simulink model "torqueWalking"  (Simulink 8.9)
settings: Solver=FixedStepDiscrete  StartTime=0.0  StopTime=Config.t_end  FixedStep=Config.t_step  RelTol=1e-3  EnableMultiTasking=on
InitFcn:
  | cd(fileparts(which(bdroot)));
  | initTorqueWalking;
StopFcn:
  | cd(fileparts(which(bdroot)));
  | outputTorqueWalking
values from neighbouring files (symbols this model uses):
  weights = [1 1 1 1 0.001 0.0001]    [inputWeights.mat]
undefined symbols (not defined in the file or in its folder): biasVectorConstraint_feet, Config, ConstraintMatrix_feet, DiscIntNeverNeededParam, Gains, ROBOT_DOF, Sat
libraries: WBToolboxLibrary x114
(part 3 of 4)

== system torqueWalking/Robot State and References/Smooth References /Smooth Reference Positions ==
  pos_CoM_des : Inport
  pos_LFoot_des : Inport  Port=2
  pos_RFoot_des : Inport  Port=3
  s_des : Inport  Port=4
  pos_LHand_des : Inport  Port=5
  pos_RHand_des : Inport  Port=6
  state : Inport  Port=7
  Configure Settling Times : MATLAB Function  TreatAsAtomicUnit=on
  Matrix Concatenate1 : Concatenate  NumInputs=3  Mode=Multidimensional array  ConcatenateDimension=2
  Matrix Concatenate{2..3,5..6} (4 alike) : Concatenate  NumInputs=4  Mode=Multidimensional array  ConcatenateDimension=2
  Matrix Concatenate4 : Concatenate  NumInputs=3  Mode=Multidimensional array  ConcatenateDimension=2
  Minimum Jerk Trajectory Generator{,1..3,5..6} (6 alike) : WBToolboxLibrary/Utilities/Minimum Jerk Trajectory Generator  externalSettlingTime=on  settlingTime=3  sampleTime=Config.t_step  resetOnSettlingTime=off  firstDerivatives=on  secondDerivatives=on  explicitInitialValue=off
  Settling time1 : Constant  Value=zeros(3,2)
  smooth_references_CoM : Outport
  smooth_pos_vel_acc_LFoot : Outport  Port=2
  smooth_pos_vel_acc_RFoot : Outport  Port=3
  smooth_pos_vel_acc_LHand : Outport  Port=4
  smooth_pos_vel_acc_RHand : Outport  Port=5
  smooth_references_s : Outport  Port=6
  wires:
  Minimum Jerk Trajectory Generator2/2 -> Matrix Concatenate3/2
  pos_RFoot_des/1 -> Minimum Jerk Trajectory Generator3/1
  s_des/1 -> Minimum Jerk Trajectory Generator1/1
  Minimum Jerk Trajectory Generator2/3 -> Matrix Concatenate3/3
  Minimum Jerk Trajectory Generator2/1 -> Matrix Concatenate3/1
  Matrix Concatenate4/1 -> smooth_references_CoM/1
  pos_CoM_des/1 -> Minimum Jerk Trajectory Generator/1
  Minimum Jerk Trajectory Generator/3 -> Matrix Concatenate4/3
  Minimum Jerk Trajectory Generator/2 -> Matrix Concatenate4/2
  Minimum Jerk Trajectory Generator3/3 -> Matrix Concatenate2/3
  Matrix Concatenate3/1 -> smooth_pos_vel_acc_LFoot/1
  Matrix Concatenate2/1 -> smooth_pos_vel_acc_RFoot/1
  Minimum Jerk Trajectory Generator/1 -> Matrix Concatenate4/1
  Minimum Jerk Trajectory Generator3/2 -> Matrix Concatenate2/2
  pos_LFoot_des/1 -> Minimum Jerk Trajectory Generator2/1
  Minimum Jerk Trajectory Generator3/1 -> Matrix Concatenate2/1
  state/1 -> Configure Settling Times/1(state)
  Configure Settling Times/1(smoothingTime_CoM) -> Minimum Jerk Trajectory Generator/2
  Configure Settling Times/2(smoothingTime_LFoot) -> Minimum Jerk Trajectory Generator2/2
  Configure Settling Times/3(smoothingTime_RFoot) -> Minimum Jerk Trajectory Generator3/2
  Configure Settling Times/4(smoothingTime_joints) -> Minimum Jerk Trajectory Generator1/2
  Configure Settling Times/6(smoothingTime_RHand) -> Minimum Jerk Trajectory Generator6/2
  Configure Settling Times/5(smoothingTime_LHand) -> Minimum Jerk Trajectory Generator5/2
  Minimum Jerk Trajectory Generator6/1 -> Matrix Concatenate5/1
  Settling time1/1 -> Matrix Concatenate3/4, Matrix Concatenate2/4, Matrix Concatenate6/4, Matrix Concatenate5/4
  Minimum Jerk Trajectory Generator6/2 -> Matrix Concatenate5/2
  Matrix Concatenate5/1 -> smooth_pos_vel_acc_RHand/1
  Matrix Concatenate6/1 -> smooth_pos_vel_acc_LHand/1
  Minimum Jerk Trajectory Generator6/3 -> Matrix Concatenate5/3
  Minimum Jerk Trajectory Generator5/1 -> Matrix Concatenate6/1
  Minimum Jerk Trajectory Generator5/3 -> Matrix Concatenate6/3
  pos_RHand_des/1 -> Minimum Jerk Trajectory Generator6/1
  pos_LHand_des/1 -> Minimum Jerk Trajectory Generator5/1
  Minimum Jerk Trajectory Generator5/2 -> Matrix Concatenate6/2
  Matrix Concatenate1/1 -> smooth_references_s/1
  Minimum Jerk Trajectory Generator1/3 -> Matrix Concatenate1/3
  Minimum Jerk Trajectory Generator1/2 -> Matrix Concatenate1/2
  Minimum Jerk Trajectory Generator1/1 -> Matrix Concatenate1/1

== system torqueWalking/Robot State and References/State Machines/Compute Feet to Base Link Transforms ==
  s : Inport
  w_H_base_fixed : Inport  Port=2
  IMU port : Inport  Port=3
  Constant : Constant  Value=Config.LFoot_in_contact_at0
  "LFoot to base link transform " : Subsystem
  LFoot to world transform (fixed base) : WBToolboxLibrary/wholeBodyModel/Kinematics/Forward Kinematics  frameName=Frames.LEFT_FOOT  robotName=WBT_robotName  localName=WBT_modelName  wbiFile=WBT_wbiFilename  wbiList=WBT_wbiList
  RFoot to base link transform : Subsystem
  RFoot to world transform (fixed base) : WBToolboxLibrary/wholeBodyModel/Kinematics/Forward Kinematics  frameName=Frames.RIGHT_FOOT  robotName=WBT_robotName  localName=WBT_modelName  wbiFile=WBT_wbiFilename  wbiList=WBT_wbiList
  Switch6 : Switch  Criteria=u2 > Threshold
  fixed_link_H_b : Outport
  LFoot_H_b : Outport  Port=2
  RFoot_H_b : Outport  Port=3
  wires:
  RFoot to world transform (fixed base)/1 -> RFoot to base link transform/3(w_H_link)
  s/1 -> RFoot to base link transform/1(s), "LFoot to base link transform "/1(s), RFoot to world transform (fixed base)/2, LFoot to world transform (fixed base)/2
  LFoot to world transform (fixed base)/1 -> "LFoot to base link transform "/3(w_H_link)
  w_H_base_fixed/1 -> RFoot to base link transform/4(w_H_base_fixed), RFoot to world transform (fixed base)/1, "LFoot to base link transform "/4(w_H_base_fixed), LFoot to world transform (fixed base)/1
  IMU port/1 -> RFoot to base link transform/2(inertial), "LFoot to base link transform "/2(inertial)
  RFoot to base link transform/1(link_H_b) -> Switch6/3, RFoot_H_b/1
  Constant/1 -> Switch6/2
  "LFoot to base link transform "/1(link_H_b) -> LFoot_H_b/1, Switch6/1
  Switch6/1 -> fixed_link_H_b/1

== system torqueWalking/Robot State and References/State Machines/Compute State Velocity ==
  s : Inport
  w_H_b : Inport  Port=2
  "feetInContact " : Inport  Port=3
  Compute Base Velocity : MATLAB Function  TreatAsAtomicUnit=on
  Feet Jacobians : Subsystem
  Get Estimate : WBToolboxLibrary/wholeBodyStates/Get Estimate  estimateType=Joints Velocity  robotName=WBT_robotName  localName=WBT_modelName  wbiFile=WBT_wbiFilename  wbiList=WBT_wbiList
  Mux : Mux  Inputs=2
  nu : Outport
  wires:
  Get Estimate/1 -> Mux/2, Compute Base Velocity/4(sDot)
  Mux/1 -> nu/1
  "feetInContact "/1 -> Compute Base Velocity/3(feetInContact)
  Compute Base Velocity/1(nu_b) -> Mux/1
  s/1 -> Feet Jacobians/1(s)
  w_H_b/1 -> Feet Jacobians/2(w_H_b)
  Feet Jacobians/1(J_LFoot) -> Compute Base Velocity/1(J_LeftFoot)
  Feet Jacobians/2(J_RFoot) -> Compute Base Velocity/2(J_RightFoot)

== system torqueWalking/Robot State and References/State Machines/Select the Current State and References ==
  s : Inport
  fixed_link_H_b : Inport  Port=2
  LFoot_H_b : Inport  Port=3
  RFoot_H_b : Inport  Port=4
  Clock : Clock
  STATE MACHINES : MATLAB Function  TreatAsAtomicUnit=on
  holder {1..7} (7 alike) : WBToolboxLibrary/Utilities/holder 
  left_foot_wrench : WBToolboxLibrary/Utilities/Yarp Read  portName=Ports.LEFT_FOOT_EXT_WRENCH  signalSize=6  blocking=off  timestamp=off  autoconnect=on  errorOnConnection=on
  right_foot_wrench : WBToolboxLibrary/Utilities/Yarp Read  portName=Ports.RIGHT_FOOT_EXT_WRENCH  signalSize=6  blocking=off  timestamp=off  autoconnect=on  errorOnConnection=on
  task position and orientation : Subsystem
  w_H_b : Outport
  feetInContact : Outport  Port=2
  state : Outport  Port=3
  references_CoM : Outport  Port=4
  references_LFoot : Outport  Port=5
  references_RFoot : Outport  Port=6
  references_rot_task : Outport  Port=7
  references_LHand : Outport  Port=8
  references_RHand : Outport  Port=9
  references_s : Outport  Port=10
  wires:
  STATE MACHINES/3(references_LFoot) -> references_LFoot/1
  task position and orientation/2(w_H_l_sole) -> holder 2/1
  holder 3/1 -> STATE MACHINES/4(w_H_RFoot_0)
  STATE MACHINES/5(references_rot_task) -> references_rot_task/1
  STATE MACHINES/4(references_RFoot) -> references_RFoot/1
  s/1 -> holder 5/1, task position and orientation/1(s)
  holder 4/1 -> STATE MACHINES/5(w_H_rot_task_0)
  task position and orientation/1(w_H_CoM) -> holder 1/1
  holder 2/1 -> STATE MACHINES/3(w_H_LFoot_0)
  task position and orientation/4(w_H_rot_task) -> holder 4/1
  STATE MACHINES/1(state) -> state/1
  STATE MACHINES/8(feetInContact) -> feetInContact/1
  task position and orientation/3(w_H_r_sole) -> holder 3/1
  Clock/1 -> STATE MACHINES/10(t)
  STATE MACHINES/9(references_s) -> references_s/1
  STATE MACHINES/2(references_CoM) -> references_CoM/1
  holder 1/1 -> STATE MACHINES/2(w_H_CoM_0)
  holder 5/1 -> STATE MACHINES/1(s_0)
  STATE MACHINES/10(w_H_b) -> w_H_b/1
  fixed_link_H_b/1 -> task position and orientation/2(w_H_b)
  LFoot_H_b/1 -> STATE MACHINES/8(LFoot_H_b)
  RFoot_H_b/1 -> STATE MACHINES/9(RFoot_H_b)
  left_foot_wrench/1 -> STATE MACHINES/11(LFoot_wrench)
  right_foot_wrench/1 -> STATE MACHINES/12(RFoot_wrench)
  holder 6/1 -> STATE MACHINES/6(w_H_LHand_0)
  task position and orientation/5(w_H_l_hand) -> holder 6/1
  task position and orientation/6(w_H_r_hand) -> holder 7/1
  holder 7/1 -> STATE MACHINES/7(w_H_RHand_0)
  STATE MACHINES/6(references_LHand) -> references_LHand/1
  STATE MACHINES/7(references_RHand) -> references_RHand/1

== system torqueWalking/Visualization/Cartesian Tasks/Rotation Error Left Foot ==
  w_R_RFoot : Inport
  w_R_RFoot_des : Inport  Port=2
  Constant : Constant  Value=eye(3)
  Demux : Demux  Outputs=3
  Permute Dimensions1 : PermuteDimensions
  Permute Dimensions2 : PermuteDimensions
  Product : Product  Multiplication=Matrix(*)
  Product2 : Product  Multiplication=Matrix(*)
  Reshape2 : Reshape
  Selector : Selector  InputPortWidth=9  IndexOptions=Index vector (dialog)  Indices=[1 5 9]  OutputSizes=1
  Sum : Sum  Inputs=|-+
  Sum of Elements : Sum  Inputs=+++
  |1-R^T*RDes|^2 : Outport
  wires:
  w_R_RFoot_des/1 -> Product2/2
  Product2/1 -> Sum/1
  w_R_RFoot/1 -> Permute Dimensions2/1
  Sum/1 -> Product/2, Permute Dimensions1/1
  Permute Dimensions2/1 -> Product2/1
  Constant/1 -> Sum/2
  Permute Dimensions1/1 -> Product/1
  Product/1 -> Reshape2/1
  Reshape2/1 -> Selector/1
  Selector/1 -> Demux/1
  Demux/1 -> Sum of Elements/1
  Demux/2 -> Sum of Elements/2
  Demux/3 -> Sum of Elements/3
  Sum of Elements/1 -> |1-R^T*RDes|^2/1

== system torqueWalking/Visualization/Cartesian Tasks/Rotation Error Right Foot ==
  w_R_LFoot : Inport
  w_R_LFoot_des : Inport  Port=2
  Constant : Constant  Value=eye(3)
  Demux : Demux  Outputs=3
  Permute Dimensions1 : PermuteDimensions
  Permute Dimensions2 : PermuteDimensions
  Product : Product  Multiplication=Matrix(*)
  Product2 : Product  Multiplication=Matrix(*)
  Reshape2 : Reshape
  Selector : Selector  InputPortWidth=9  IndexOptions=Index vector (dialog)  Indices=[1 5 9]  OutputSizes=1
  Sum : Sum  Inputs=|-+
  Sum of Elements : Sum  Inputs=+++
  |1-R^T*RDes|^2 : Outport
  wires:
  w_R_LFoot_des/1 -> Product2/2
  Product2/1 -> Sum/1
  w_R_LFoot/1 -> Permute Dimensions2/1
  Sum/1 -> Product/2, Permute Dimensions1/1
  Permute Dimensions2/1 -> Product2/1
  Constant/1 -> Sum/2
  Permute Dimensions1/1 -> Product/1
  Product/1 -> Reshape2/1
  Reshape2/1 -> Selector/1
  Selector/1 -> Demux/1
  Demux/1 -> Sum of Elements/1
  Demux/2 -> Sum of Elements/2
  Demux/3 -> Sum of Elements/3
  Sum of Elements/1 -> |1-R^T*RDes|^2/1

== system torqueWalking/Visualization/Cartesian Tasks/Rotation Error Rotational Task ==
  w_R_rot_task : Inport
  w_R_rot_task_des : Inport  Port=2
  Constant : Constant  Value=eye(3)
  Demux : Demux  Outputs=3
  Permute Dimensions1 : PermuteDimensions
  Permute Dimensions2 : PermuteDimensions
  Product : Product  Multiplication=Matrix(*)
  Product2 : Product  Multiplication=Matrix(*)
  Reshape2 : Reshape
  Selector : Selector  InputPortWidth=9  IndexOptions=Index vector (dialog)  Indices=[1 5 9]  OutputSizes=1
  Sum : Sum  Inputs=|-+
  Sum of Elements : Sum  Inputs=+++
  |1-R^T*RDes|^2 : Outport
  wires:
  w_R_rot_task_des/1 -> Product2/2
  Product2/1 -> Sum/1
  w_R_rot_task/1 -> Permute Dimensions2/1
  Sum/1 -> Product/2, Permute Dimensions1/1
  Permute Dimensions2/1 -> Product2/1
  Constant/1 -> Sum/2
  Permute Dimensions1/1 -> Product/1
  Product/1 -> Reshape2/1
  Reshape2/1 -> Selector/1
  Selector/1 -> Demux/1
  Demux/1 -> Sum of Elements/1
  Demux/2 -> Sum of Elements/2
  Demux/3 -> Sum of Elements/3
  Sum of Elements/1 -> |1-R^T*RDes|^2/1

== system torqueWalking/Visualization/Orientation Tasks References/Rotation Error Left Foot ==
  w_R_LFoot : Inport
  w_R_LFoot_des : Inport  Port=2
  Constant : Constant  Value=eye(3)
  Demux : Demux  Outputs=3
  Permute Dimensions1 : PermuteDimensions
  Permute Dimensions2 : PermuteDimensions
  Product : Product  Multiplication=Matrix(*)
  Product2 : Product  Multiplication=Matrix(*)
  Reshape2 : Reshape
  Selector : Selector  InputPortWidth=9  IndexOptions=Index vector (dialog)  Indices=[1 5 9]  OutputSizes=1
  Sum : Sum  Inputs=|-+
  Sum of Elements : Sum  Inputs=+++
  |1-R^T*RDes|^2 : Outport
  wires:
  w_R_LFoot_des/1 -> Product2/2
  Product2/1 -> Sum/1
  w_R_LFoot/1 -> Permute Dimensions2/1
  Sum/1 -> Product/2, Permute Dimensions1/1
  Permute Dimensions2/1 -> Product2/1
  Constant/1 -> Sum/2
  Permute Dimensions1/1 -> Product/1
  Product/1 -> Reshape2/1
  Reshape2/1 -> Selector/1
  Selector/1 -> Demux/1
  Demux/1 -> Sum of Elements/1
  Demux/2 -> Sum of Elements/2
  Demux/3 -> Sum of Elements/3
  Sum of Elements/1 -> |1-R^T*RDes|^2/1

== system torqueWalking/Visualization/Orientation Tasks References/Rotation Error Right Foot ==
  w_R_RFoot : Inport
  w_R_RFoot_des : Inport  Port=2
  Constant : Constant  Value=eye(3)
  Demux : Demux  Outputs=3
  Permute Dimensions1 : PermuteDimensions
  Permute Dimensions2 : PermuteDimensions
  Product : Product  Multiplication=Matrix(*)
  Product2 : Product  Multiplication=Matrix(*)
  Reshape2 : Reshape
  Selector : Selector  InputPortWidth=9  IndexOptions=Index vector (dialog)  Indices=[1 5 9]  OutputSizes=1
  Sum : Sum  Inputs=|-+
  Sum of Elements : Sum  Inputs=+++
  |1-R^T*RDes|^2 : Outport
  wires:
  w_R_RFoot_des/1 -> Product2/2
  Product2/1 -> Sum/1
  w_R_RFoot/1 -> Permute Dimensions2/1
  Sum/1 -> Product/2, Permute Dimensions1/1
  Permute Dimensions2/1 -> Product2/1
  Constant/1 -> Sum/2
  Permute Dimensions1/1 -> Product/1
  Product/1 -> Reshape2/1
  Reshape2/1 -> Selector/1
  Selector/1 -> Demux/1
  Demux/1 -> Sum of Elements/1
  Demux/2 -> Sum of Elements/2
  Demux/3 -> Sum of Elements/3
  Sum of Elements/1 -> |1-R^T*RDes|^2/1

== system torqueWalking/Visualization/Orientation Tasks References/Rotation Error Rotational Task ==
  w_R_rot_task : Inport
  w_R_rot_task_des : Inport  Port=2
  Constant : Constant  Value=eye(3)
  Demux : Demux  Outputs=3
  Permute Dimensions1 : PermuteDimensions
  Permute Dimensions2 : PermuteDimensions
  Product : Product  Multiplication=Matrix(*)
  Product2 : Product  Multiplication=Matrix(*)
  Reshape2 : Reshape
  Selector : Selector  InputPortWidth=9  IndexOptions=Index vector (dialog)  Indices=[1 5 9]  OutputSizes=1
  Sum : Sum  Inputs=|-+
  Sum of Elements : Sum  Inputs=+++
  |1-R^T*RDes|^2 : Outport
  wires:
  w_R_rot_task_des/1 -> Product2/2
  Product2/1 -> Sum/1
  w_R_rot_task/1 -> Permute Dimensions2/1
  Sum/1 -> Product/2, Permute Dimensions1/1
  Permute Dimensions2/1 -> Product2/1
  Constant/1 -> Sum/2
  Permute Dimensions1/1 -> Product/1
  Product/1 -> Reshape2/1
  Reshape2/1 -> Selector/1
  Selector/1 -> Demux/1
  Demux/1 -> Sum of Elements/1
  Demux/2 -> Sum of Elements/2
  Demux/3 -> Sum of Elements/3
  Sum of Elements/1 -> |1-R^T*RDes|^2/1

== system torqueWalking/Dynamics and Kinematics/Compute Dynamic and Kinematic Quantities/Mass Matrix and Bias Forces/Add motors reflected inertias ==
  M : Inport
  Add motor reflected inertias : MATLAB Function  TreatAsAtomicUnit=on
  M_with_motor_inertia : Outport
  wires:
  M/1 -> Add motor reflected inertias/1(M)
  Add motor reflected inertias/1(M_with_inertia) -> M_with_motor_inertia/1

== system torqueWalking/Dynamics and Kinematics/Initial Conditions/compute state velocity/Feet Jacobians ==
  s : Inport
  w_H_b : Inport  Port=2
  Jacobian LFoot : WBToolboxLibrary/wholeBodyModel/Jacobians/Jacobian  frameName=Frames.LEFT_FOOT  robotName=WBT_robotName  localName=WBT_modelName  wbiFile=WBT_wbiFilename  wbiList=WBT_wbiList
  Jacobian RFoot : WBToolboxLibrary/wholeBodyModel/Jacobians/Jacobian  frameName=Frames.RIGHT_FOOT  robotName=WBT_robotName  localName=WBT_modelName  wbiFile=WBT_wbiFilename  wbiList=WBT_wbiList
  J_LFoot : Outport
  J_RFoot : Outport  Port=2
  wires:
  Jacobian LFoot/1 -> J_LFoot/1
  Jacobian RFoot/1 -> J_RFoot/1
  w_H_b/1 -> Jacobian RFoot/1, Jacobian LFoot/1
  s/1 -> Jacobian LFoot/2, Jacobian RFoot/2

== system torqueWalking/Dynamics and Kinematics/Inverse Kinematics/ComputeTasksPoseAndVelocity/Task position and orientation ==
  s : Inport
  w_H_b : Inport  Port=2
  CoM : WBToolboxLibrary/wholeBodyModel/Kinematics/Forward Kinematics  frameName=Frames.COM  robotName=WBT_robotName  localName=WBT_modelName  wbiFile=WBT_wbiFilename  wbiList=WBT_wbiList
  LFoot : WBToolboxLibrary/wholeBodyModel/Kinematics/Forward Kinematics  frameName=Frames.LEFT_FOOT  robotName=WBT_robotName  localName=WBT_modelName  wbiFile=WBT_wbiFilename  wbiList=WBT_wbiList
  LFoot1 : WBToolboxLibrary/wholeBodyModel/Kinematics/Forward Kinematics  frameName=Frames.LEFT_HAND  robotName=WBT_robotName  localName=WBT_modelName  wbiFile=WBT_wbiFilename  wbiList=WBT_wbiList
  RFoot : WBToolboxLibrary/wholeBodyModel/Kinematics/Forward Kinematics  frameName=Frames.RIGHT_FOOT  robotName=WBT_robotName  localName=WBT_modelName  wbiFile=WBT_wbiFilename  wbiList=WBT_wbiList
  RFoot1 : WBToolboxLibrary/wholeBodyModel/Kinematics/Forward Kinematics  frameName=Frames.RIGHT_HAND  robotName=WBT_robotName  localName=WBT_modelName  wbiFile=WBT_wbiFilename  wbiList=WBT_wbiList
  rotational task : WBToolboxLibrary/wholeBodyModel/Kinematics/Forward Kinematics  frameName=Frames.ROT_TASK_LINK  robotName=WBT_robotName  localName=WBT_modelName  wbiFile=WBT_wbiFilename  wbiList=WBT_wbiList
  w_H_CoM : Outport
  w_H_l_sole : Outport  Port=2
  w_H_r_sole : Outport  Port=3
  w_H_rot_task : Outport  Port=4
  w_H_l_hand : Outport  Port=5
  w_H_r_hand : Outport  Port=6
  wires:
  s/1 -> rotational task/2, RFoot1/2, LFoot1/2, RFoot/2, LFoot/2, CoM/2
  w_H_b/1 -> LFoot1/1, RFoot1/1, rotational task/1, CoM/1, LFoot/1, RFoot/1
  CoM/1 -> w_H_CoM/1
  LFoot/1 -> w_H_l_sole/1
  RFoot/1 -> w_H_r_sole/1
  rotational task/1 -> w_H_rot_task/1
  RFoot1/1 -> w_H_r_hand/1
  LFoot1/1 -> w_H_l_hand/1

== system torqueWalking/Dynamics and Kinematics/Inverse Kinematics/QP-Based Inverse Kinematics/QP Solver (inverse kinematics) ==
  Hessian : Inport
  gradient : Inport  Port=2
  ConstraintMatrix : Inport  Port=3
  biasVectorConstraint : Inport  Port=4
  QPSolver : M-S-Function  FunctionName=QPInverseKinematics  Parameters=ROBOT_DOF, Sat, Config
  nuDot : Outport
  ExitFlagQP : Outport  Port=2
  wires:
  QPSolver/1 -> nuDot/1
  QPSolver/2 -> ExitFlagQP/1
  Hessian/1 -> QPSolver/1
  gradient/1 -> QPSolver/2
  biasVectorConstraint/1 -> QPSolver/4
  ConstraintMatrix/1 -> QPSolver/3

== system torqueWalking/Dynamics and Kinematics/Inverse Kinematics/QP-Based Inverse Kinematics/inverse kinematics integration ==
  nuDot : Inport
  nu_0 : Inport  Port=2
  q_0 : Inport  Port=3
  Compute Base Pose Derivative : MATLAB Function  TreatAsAtomicUnit=on
  Demux : Demux  Outputs=[7;ROBOT_DOF]
  Demux1 : Demux  Outputs=[6; ROBOT_DOF]
  Demux2 : Demux  Outputs=[16; ROBOT_DOF]
  Integrate nu : DiscreteIntegrator  InitialConditionSource=external  SampleTime=Config.t_step  ICPrevOutput=DiscIntNeverNeededParam  ICPrevScaledInput=DiscIntNeverNeededParam
  Integrate nuDot : DiscreteIntegrator  InitialConditionSource=external  SampleTime=Config.t_step  ICPrevOutput=DiscIntNeverNeededParam  ICPrevScaledInput=DiscIntNeverNeededParam
  Matrix Concatenate : Concatenate  NumInputs=3  Mode=Multidimensional array  ConcatenateDimension=2
  Mux : Mux  Inputs=2
  Mux1 : Mux  Inputs=2
  Mux2 : Mux  Inputs=2
  Reshape : Reshape
  Reshape1 : Reshape  OutputDimensionality=Customize  OutputDimensions=[4;4]
  Rewrite Base Pose as pos+quat : MATLAB Function  TreatAsAtomicUnit=on
  Rewrite Base Pose as transformation matrix : MATLAB Function  TreatAsAtomicUnit=on
  Selector3 : Selector  InputPortWidth=ROBOT_DOF+6  IndexOptions=Index vector (dialog)  Indices=[7:ROBOT_DOF+6]  OutputSizes=1
  Selector4 : Selector  InputPortWidth=ROBOT_DOF+6  IndexOptions=Index vector (dialog)  Indices=[7:ROBOT_DOF+6]  OutputSizes=1
  nu : Outport
  q : Outport  Port=2
  s_sDot_sDDot_des : Outport  Port=3
  wires:
  nu_0/1 -> Integrate nuDot/2
  nuDot/1 -> Selector4/1, Integrate nuDot/1
  Demux/1 -> Rewrite Base Pose as transformation matrix/1(pose_b), Compute Base Pose Derivative/1(pose_b)
  Integrate nu/1 -> Demux/1
  Compute Base Pose Derivative/1(pose_bDot) -> Mux/1
  Demux1/2 -> Mux/2
  Matrix Concatenate/1 -> s_sDot_sDDot_des/1
  Selector3/1 -> Matrix Concatenate/2
  Selector4/1 -> Matrix Concatenate/3
  Demux/2 -> Matrix Concatenate/1, Mux1/2
  Mux/1 -> Integrate nu/1
  Integrate nuDot/1 -> Selector3/1, nu/1, Demux1/1
  Rewrite Base Pose as transformation matrix/1(w_H_b) -> Reshape/1
  Reshape/1 -> Mux1/1
  Mux1/1 -> q/1
  Demux1/1 -> Compute Base Pose Derivative/2(nu_b)
  q_0/1 -> Demux2/1
  Demux2/1 -> Reshape1/1
  Reshape1/1 -> Rewrite Base Pose as pos+quat/1(w_H_b_0)
  Rewrite Base Pose as pos+quat/1(pose_b_0) -> Mux2/1
  Demux2/2 -> Mux2/2
  Mux2/1 -> Integrate nu/2

== system torqueWalking/Dynamics and Kinematics/Task Accelerations/ComputeTasksPoseAndVelocity/Task position and orientation ==
  s : Inport
  w_H_b : Inport  Port=2
  CoM : WBToolboxLibrary/wholeBodyModel/Kinematics/Forward Kinematics  frameName=Frames.COM  robotName=WBT_robotName  localName=WBT_modelName  wbiFile=WBT_wbiFilename  wbiList=WBT_wbiList
  LFoot : WBToolboxLibrary/wholeBodyModel/Kinematics/Forward Kinematics  frameName=Frames.LEFT_FOOT  robotName=WBT_robotName  localName=WBT_modelName  wbiFile=WBT_wbiFilename  wbiList=WBT_wbiList
  LHand : WBToolboxLibrary/wholeBodyModel/Kinematics/Forward Kinematics  frameName=Frames.LEFT_FOOT  robotName=WBT_robotName  localName=WBT_modelName  wbiFile=WBT_wbiFilename  wbiList=WBT_wbiList
  RFoot : WBToolboxLibrary/wholeBodyModel/Kinematics/Forward Kinematics  frameName=Frames.RIGHT_FOOT  robotName=WBT_robotName  localName=WBT_modelName  wbiFile=WBT_wbiFilename  wbiList=WBT_wbiList
  RHand : WBToolboxLibrary/wholeBodyModel/Kinematics/Forward Kinematics  frameName=Frames.RIGHT_FOOT  robotName=WBT_robotName  localName=WBT_modelName  wbiFile=WBT_wbiFilename  wbiList=WBT_wbiList
  rotational task : WBToolboxLibrary/wholeBodyModel/Kinematics/Forward Kinematics  frameName=Frames.ROT_TASK_LINK  robotName=WBT_robotName  localName=WBT_modelName  wbiFile=WBT_wbiFilename  wbiList=WBT_wbiList
  w_H_CoM : Outport
  w_H_l_sole : Outport  Port=2
  w_H_r_sole : Outport  Port=3
  w_H_rot_task : Outport  Port=4
  w_H_l_hand : Outport  Port=5
  w_H_r_hand : Outport  Port=6
  wires:
  s/1 -> RHand/2, LHand/2, rotational task/2, RFoot/2, LFoot/2, CoM/2
  w_H_b/1 -> RHand/1, LHand/1, rotational task/1, CoM/1, LFoot/1, RFoot/1
  CoM/1 -> w_H_CoM/1
  LFoot/1 -> w_H_l_sole/1
  RFoot/1 -> w_H_r_sole/1
  rotational task/1 -> w_H_rot_task/1
  RHand/1 -> w_H_r_hand/1
  LHand/1 -> w_H_l_hand/1

== system torqueWalking/Robot State and References/Smooth References /Smooth Reference Orientations/Compose Smoothed References ==
  omegaDot_LFoot : Inport
  omegaDot_RFoot : Inport  Port=2
  omegaDot_rot_task : Inport  Port=3
  omegaDot_LHand : Inport  Port=4
  omegaDot_RHand : Inport  Port=5
  w_R_RHand : Inport  Port=6
  w_R_LHand : Inport  Port=7
  w_R_rot_task : Inport  Port=8
  w_R_RFoot : Inport  Port=9
  w_R_LFoot : Inport  Port=10
  omega_LFoot : Inport  Port=11
  omega_RFoot : Inport  Port=12
  omega_rot_task : Inport  Port=13
  omega_LHand : Inport  Port=14
  omega_RHand : Inport  Port=15
  Matrix Concatenate{1..4,6} (5 alike) : Concatenate  NumInputs=3  Mode=Multidimensional array  ConcatenateDimension=2
  orient_vel_acc_LFoot_des : Outport
  orient_vel_acc_RFoot_des : Outport  Port=2
  orient_vel_acc_rot_task_des : Outport  Port=3
  orient_vel_acc_LHand_des : Outport  Port=4
  orient_vel_acc_RHand_des : Outport  Port=5
  wires:
  w_R_LFoot/1 -> Matrix Concatenate6/1
  Matrix Concatenate6/1 -> orient_vel_acc_LFoot_des/1
  Matrix Concatenate2/1 -> orient_vel_acc_rot_task_des/1
  Matrix Concatenate1/1 -> orient_vel_acc_RFoot_des/1
  omega_LFoot/1 -> Matrix Concatenate6/2
  omegaDot_LFoot/1 -> Matrix Concatenate6/3
  omegaDot_RFoot/1 -> Matrix Concatenate1/3
  omega_RFoot/1 -> Matrix Concatenate1/2
  w_R_RFoot/1 -> Matrix Concatenate1/1
  omegaDot_rot_task/1 -> Matrix Concatenate2/3
  omega_rot_task/1 -> Matrix Concatenate2/2
  w_R_rot_task/1 -> Matrix Concatenate2/1
  w_R_RHand/1 -> Matrix Concatenate3/1
  omega_RHand/1 -> Matrix Concatenate3/2
  omegaDot_RHand/1 -> Matrix Concatenate3/3
  omegaDot_LHand/1 -> Matrix Concatenate4/3
  omega_LHand/1 -> Matrix Concatenate4/2
  Matrix Concatenate3/1 -> orient_vel_acc_RHand_des/1
  Matrix Concatenate4/1 -> orient_vel_acc_LHand_des/1
  w_R_LHand/1 -> Matrix Concatenate4/1

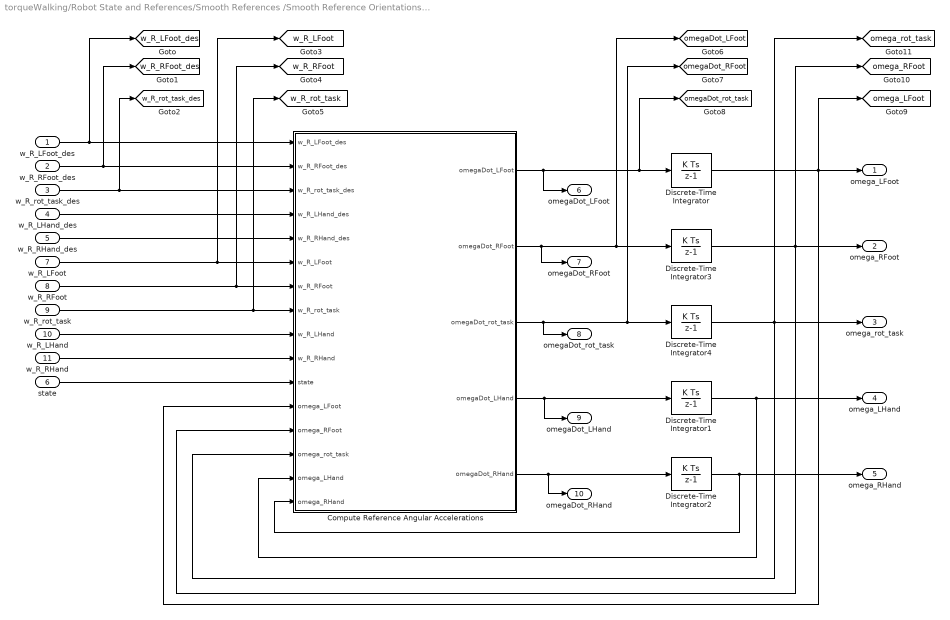
== system torqueWalking/Robot State and References/Smooth References /Smooth Reference Orientations/Compute Ref Ang Velocities and Accelerations ==
  w_R_LFoot_des : Inport
  w_R_RFoot_des : Inport  Port=2
  w_R_rot_task_des : Inport  Port=3
  w_R_LHand_des : Inport  Port=4
  w_R_RHand_des : Inport  Port=5
  state : Inport  Port=6
  w_R_LFoot : Inport  Port=7
  w_R_RFoot : Inport  Port=8
  w_R_rot_task : Inport  Port=9
  w_R_LHand : Inport  Port=10
  w_R_RHand : Inport  Port=11
  Compute Reference Angular Accelerations : MATLAB Function  TreatAsAtomicUnit=on
  Discrete-Time Integrator{,1..4} (5 alike) : DiscreteIntegrator  InitialCondition=zeros(3,1)  InitialConditionSetting=State (most efficient)  SampleTime=Config.t_step  ICPrevOutput=DiscIntNeverNeededParam  ICPrevScaledInput=DiscIntNeverNeededParam
  omega_LFoot : Outport
  omega_RFoot : Outport  Port=2
  omega_rot_task : Outport  Port=3
  omega_LHand : Outport  Port=4
  omega_RHand : Outport  Port=5
  omegaDot_LFoot : Outport  Port=6
  omegaDot_RFoot : Outport  Port=7
  omegaDot_rot_task : Outport  Port=8
  omegaDot_LHand : Outport  Port=9
  omegaDot_RHand : Outport  Port=10
  tag scope: omegaDot_LFoot=global, omegaDot_RFoot=global, omegaDot_rot_task=global, omega_LFoot=global, omega_RFoot=global, omega_rot_task=global, w_R_LFoot=global, w_R_LFoot_des=global, w_R_RFoot=global, w_R_RFoot_des=global, w_R_rot_task=global, w_R_rot_task_des=global
  wires:
  w_R_RFoot/1 -> [w_R_RFoot], Compute Reference Angular Accelerations/7(w_R_RFoot)
  w_R_rot_task/1 -> [w_R_rot_task], Compute Reference Angular Accelerations/8(w_R_rot_task)
  w_R_LFoot/1 -> [w_R_LFoot], Compute Reference Angular Accelerations/6(w_R_LFoot)
  Compute Reference Angular Accelerations/1(omegaDot_LFoot) -> [omegaDot_rot_task], Discrete-Time Integrator/1, omegaDot_LFoot/1
  Compute Reference Angular Accelerations/3(omegaDot_rot_task) -> omegaDot_rot_task/1, [omegaDot_RFoot], Discrete-Time Integrator4/1
  Compute Reference Angular Accelerations/2(omegaDot_RFoot) -> omegaDot_RFoot/1, Discrete-Time Integrator3/1, [omegaDot_LFoot]
  w_R_LFoot_des/1 -> [w_R_LFoot_des], Compute Reference Angular Accelerations/1(w_R_LFoot_des)
  w_R_RFoot_des/1 -> [w_R_RFoot_des], Compute Reference Angular Accelerations/2(w_R_RFoot_des)
  w_R_rot_task_des/1 -> [w_R_rot_task_des], Compute Reference Angular Accelerations/3(w_R_rot_task_des)
  state/1 -> Compute Reference Angular Accelerations/11(state)
  Discrete-Time Integrator4/1 -> Compute Reference Angular Accelerations/14(omega_rot_task), omega_rot_task/1, [omega_rot_task]
  Discrete-Time Integrator3/1 -> Compute Reference Angular Accelerations/13(omega_RFoot), omega_RFoot/1, [omega_RFoot]
  Discrete-Time Integrator/1 -> [omega_LFoot], Compute Reference Angular Accelerations/12(omega_LFoot), omega_LFoot/1
  w_R_RHand/1 -> Compute Reference Angular Accelerations/10(w_R_RHand)
  w_R_LHand/1 -> Compute Reference Angular Accelerations/9(w_R_LHand)
  Discrete-Time Integrator1/1 -> Compute Reference Angular Accelerations/15(omega_LHand), omega_LHand/1
  Discrete-Time Integrator2/1 -> Compute Reference Angular Accelerations/16(omega_RHand), omega_RHand/1
  Compute Reference Angular Accelerations/4(omegaDot_LHand) -> omegaDot_LHand/1, Discrete-Time Integrator1/1
  Compute Reference Angular Accelerations/5(omegaDot_RHand) -> omegaDot_RHand/1, Discrete-Time Integrator2/1
  w_R_LHand_des/1 -> Compute Reference Angular Accelerations/4(w_R_LHand_des)
  w_R_RHand_des/1 -> Compute Reference Angular Accelerations/5(w_R_RHand_des)

== system torqueWalking/Robot State and References/Smooth References /Smooth Reference Orientations/Compute Smoothed Ref Orientations ==
  w_R_LFoot_des : Inport
  w_R_RFoot_des : Inport  Port=2
  w_R_rot_task_des : Inport  Port=3
  w_R_LHand_des : Inport  Port=4
  w_R_RHand_des : Inport  Port=5
  omega_LFoot : Inport  Port=6
  omega_RFoot : Inport  Port=7
  omega_rot_task : Inport  Port=8
  omega_LHand : Inport  Port=9
  omega_RHand : Inport  Port=10
  Compute Rotation Matrix Derivative : MATLAB Function  TreatAsAtomicUnit=on
  Discrete-Time Integrator{1..5} (5 alike) : DiscreteIntegrator  InitialConditionSource=external  InitialCondition=zeros(3,1)  InitialConditionSetting=State (most efficient)  SampleTime=Config.t_step  ICPrevOutput=DiscIntNeverNeededParam  ICPrevScaledInput=DiscIntNeverNeededParam
  holder {,1..4} (5 alike) : WBToolboxLibrary/Utilities/holder 
  w_R_LFoot : Outport
  w_R_RFoot : Outport  Port=2
  w_R_rot_task : Outport  Port=3
  w_R_LHand : Outport  Port=4
  w_R_RHand : Outport  Port=5
  wires:
  "holder "/1 -> Discrete-Time Integrator2/2
  holder 2/1 -> Discrete-Time Integrator5/2
  holder 1/1 -> Discrete-Time Integrator1/2
  Compute Rotation Matrix Derivative/1(RDot_LFoot) -> Discrete-Time Integrator2/1
  Compute Rotation Matrix Derivative/2(RDot_RFoot) -> Discrete-Time Integrator5/1
  Compute Rotation Matrix Derivative/3(RDot_rot_task) -> Discrete-Time Integrator1/1
  w_R_LFoot_des/1 -> "holder "/1
  w_R_RFoot_des/1 -> holder 2/1
  w_R_rot_task_des/1 -> holder 1/1
  Discrete-Time Integrator2/1 -> w_R_LFoot/1, Compute Rotation Matrix Derivative/6(w_R_LFoot)
  Discrete-Time Integrator1/1 -> w_R_rot_task/1, Compute Rotation Matrix Derivative/8(w_R_rot_task)
  omega_LFoot/1 -> Compute Rotation Matrix Derivative/1(omega_LFoot)
  omega_RFoot/1 -> Compute Rotation Matrix Derivative/2(omega_RFoot)
  omega_rot_task/1 -> Compute Rotation Matrix Derivative/3(omega_rot_task)
  Discrete-Time Integrator5/1 -> w_R_RFoot/1, Compute Rotation Matrix Derivative/7(w_R_RFoot)
  omega_LHand/1 -> Compute Rotation Matrix Derivative/4(omega_LHand)
  omega_RHand/1 -> Compute Rotation Matrix Derivative/5(omega_RHand)
  Discrete-Time Integrator4/1 -> w_R_RHand/1, Compute Rotation Matrix Derivative/10(w_R_RHand)
  Discrete-Time Integrator3/1 -> w_R_LHand/1, Compute Rotation Matrix Derivative/9(w_R_LHand)
  w_R_RHand_des/1 -> holder 4/1
  w_R_LHand_des/1 -> holder 3/1
  Compute Rotation Matrix Derivative/5(RDot_RHand) -> Discrete-Time Integrator4/1
  Compute Rotation Matrix Derivative/4(RDot_LHand) -> Discrete-Time Integrator3/1
  holder 4/1 -> Discrete-Time Integrator4/2
  holder 3/1 -> Discrete-Time Integrator3/2

== system torqueWalking/Robot State and References/State Machines/Compute Feet to Base Link Transforms/LFoot to base link transform  ==
  s : Inport
  inertial : Inport  Port=2
  w_H_link : Inport  Port=3
  w_H_base_fixed : Inport  Port=4
  Fixed base to imu transform : WBToolboxLibrary/wholeBodyModel/Kinematics/Forward Kinematics  frameName=Frames.IMU  robotName=WBT_robotName  localName=WBT_modelName  wbiFile=WBT_wbiFilename  wbiList=WBT_wbiList
  Fixed base to root link transform : WBToolboxLibrary/wholeBodyModel/Kinematics/Forward Kinematics  frameName=Frames.BASE_LINK  robotName=WBT_robotName  localName=WBT_modelName  wbiFile=WBT_wbiFilename  wbiList=WBT_wbiList
  Inv\* : Product  Inputs=/*  Multiplication=Matrix(*)
  "Inv\\*  " : Product  Inputs=/*  Multiplication=Matrix(*)
  Neck Position : WBToolboxLibrary/Utilities/Yarp Read  portName=Ports.NECK_POS  signalSize=6  blocking=off  timestamp=off  autoconnect=on  errorOnConnection=off
  Switch6 : Switch  Criteria=u2 > Threshold
  USE_IMU4EST_BASE : Constant  Value=Config.USE_IMU4EST_BASE
  fromImuToHomogeousTransformFCN : MATLAB Function  TreatAsAtomicUnit=on
  holder 1 : WBToolboxLibrary/Utilities/holder 
  holder 2 : WBToolboxLibrary/Utilities/holder 
  neck transform : Subsystem
  link_H_b : Outport
  wires:
  Switch6/1 -> link_H_b/1
  "Inv\\*  "/1 -> Switch6/3, fromImuToHomogeousTransformFCN/3(link_H_base)  "link_H_root"
  USE_IMU4EST_BASE/1 -> Switch6/2
  Inv\*/1 -> fromImuToHomogeousTransformFCN/1(imu_H_link), holder 1/1  "imu_H_link"
  holder 2/1 -> fromImuToHomogeousTransformFCN/4(inertial_0)
  Fixed base to imu transform/1 -> Inv\*/1
  holder 1/1 -> fromImuToHomogeousTransformFCN/2(imu_H_link_0)
  s/1 -> Fixed base to imu transform/2, Fixed base to root link transform/2
  fromImuToHomogeousTransformFCN/1(w_H_b) -> Switch6/1
  Fixed base to root link transform/1 -> "Inv\\*  "/2
  inertial/1 -> holder 2/1, fromImuToHomogeousTransformFCN/5(inertial)
  Neck Position/1 -> neck transform/1(neck port)
  neck transform/1(neck position) -> fromImuToHomogeousTransformFCN/6(neck_pos)
  w_H_link/1 -> "Inv\\*  "/1, Inv\*/2
  w_H_base_fixed/1 -> Fixed base to root link transform/1, Fixed base to imu transform/1

== system torqueWalking/Robot State and References/State Machines/Compute Feet to Base Link Transforms/RFoot to base link transform ==
  s : Inport
  inertial : Inport  Port=2
  w_H_link : Inport  Port=3
  w_H_base_fixed : Inport  Port=4
  Fixed base to imu transform : WBToolboxLibrary/wholeBodyModel/Kinematics/Forward Kinematics  frameName=Frames.IMU  robotName=WBT_robotName  localName=WBT_modelName  wbiFile=WBT_wbiFilename  wbiList=WBT_wbiList
  Fixed base to root link transform : WBToolboxLibrary/wholeBodyModel/Kinematics/Forward Kinematics  frameName=Frames.BASE_LINK  robotName=WBT_robotName  localName=WBT_modelName  wbiFile=WBT_wbiFilename  wbiList=WBT_wbiList
  Inv\* : Product  Inputs=/*  Multiplication=Matrix(*)
  "Inv\\*  " : Product  Inputs=/*  Multiplication=Matrix(*)
  Neck Position : WBToolboxLibrary/Utilities/Yarp Read  portName=Ports.NECK_POS  signalSize=6  blocking=off  timestamp=off  autoconnect=on  errorOnConnection=off
  Switch6 : Switch  Criteria=u2 > Threshold
  USE_IMU4EST_BASE : Constant  Value=Config.USE_IMU4EST_BASE
  fromImuToHomogeousTransformFCN : MATLAB Function  TreatAsAtomicUnit=on
  holder 1 : WBToolboxLibrary/Utilities/holder 
  holder 2 : WBToolboxLibrary/Utilities/holder 
  neck transform : Subsystem
  link_H_b : Outport
  wires:
  Switch6/1 -> link_H_b/1
  "Inv\\*  "/1 -> Switch6/3, fromImuToHomogeousTransformFCN/3(link_H_base)  "link_H_root"
  USE_IMU4EST_BASE/1 -> Switch6/2
  Inv\*/1 -> fromImuToHomogeousTransformFCN/1(imu_H_link), holder 1/1  "imu_H_link"
  holder 2/1 -> fromImuToHomogeousTransformFCN/4(inertial_0)
  Fixed base to imu transform/1 -> Inv\*/1
  holder 1/1 -> fromImuToHomogeousTransformFCN/2(imu_H_link_0)
  s/1 -> Fixed base to imu transform/2, Fixed base to root link transform/2
  fromImuToHomogeousTransformFCN/1(w_H_b) -> Switch6/1
  Fixed base to root link transform/1 -> "Inv\\*  "/2
  inertial/1 -> holder 2/1, fromImuToHomogeousTransformFCN/5(inertial)
  Neck Position/1 -> neck transform/1(neck port)
  neck transform/1(neck position) -> fromImuToHomogeousTransformFCN/6(neck_pos)
  w_H_link/1 -> "Inv\\*  "/1, Inv\*/2
  w_H_base_fixed/1 -> Fixed base to root link transform/1, Fixed base to imu transform/1

== system torqueWalking/Robot State and References/State Machines/Compute State Velocity/Feet Jacobians ==
  s : Inport
  w_H_b : Inport  Port=2
  Jacobian LFoot : WBToolboxLibrary/wholeBodyModel/Jacobians/Jacobian  frameName=Frames.LEFT_FOOT  robotName=WBT_robotName  localName=WBT_modelName  wbiFile=WBT_wbiFilename  wbiList=WBT_wbiList
  Jacobian RFoot : WBToolboxLibrary/wholeBodyModel/Jacobians/Jacobian  frameName=Frames.RIGHT_FOOT  robotName=WBT_robotName  localName=WBT_modelName  wbiFile=WBT_wbiFilename  wbiList=WBT_wbiList
  J_LFoot : Outport
  J_RFoot : Outport  Port=2
  wires:
  Jacobian LFoot/1 -> J_LFoot/1
  Jacobian RFoot/1 -> J_RFoot/1
  w_H_b/1 -> Jacobian RFoot/1, Jacobian LFoot/1
  s/1 -> Jacobian LFoot/2, Jacobian RFoot/2

== system torqueWalking/Robot State and References/State Machines/Select the Current State and References/task position and orientation ==
  s : Inport
  w_H_b : Inport  Port=2
  CoM : WBToolboxLibrary/wholeBodyModel/Kinematics/Forward Kinematics  frameName=Frames.COM  robotName=WBT_robotName  localName=WBT_modelName  wbiFile=WBT_wbiFilename  wbiList=WBT_wbiList
  LArm : WBToolboxLibrary/wholeBodyModel/Kinematics/Forward Kinematics  frameName=Frames.LEFT_HAND  robotName=WBT_robotName  localName=WBT_modelName  wbiFile=WBT_wbiFilename  wbiList=WBT_wbiList
  LFoot : WBToolboxLibrary/wholeBodyModel/Kinematics/Forward Kinematics  frameName=Frames.LEFT_FOOT  robotName=WBT_robotName  localName=WBT_modelName  wbiFile=WBT_wbiFilename  wbiList=WBT_wbiList
  RArm : WBToolboxLibrary/wholeBodyModel/Kinematics/Forward Kinematics  frameName=Frames.RIGHT_HAND  robotName=WBT_robotName  localName=WBT_modelName  wbiFile=WBT_wbiFilename  wbiList=WBT_wbiList
  RFoot : WBToolboxLibrary/wholeBodyModel/Kinematics/Forward Kinematics  frameName=Frames.RIGHT_FOOT  robotName=WBT_robotName  localName=WBT_modelName  wbiFile=WBT_wbiFilename  wbiList=WBT_wbiList
  rotational task : WBToolboxLibrary/wholeBodyModel/Kinematics/Forward Kinematics  frameName=Frames.ROT_TASK_LINK  robotName=WBT_robotName  localName=WBT_modelName  wbiFile=WBT_wbiFilename  wbiList=WBT_wbiList
  w_H_CoM : Outport
  w_H_l_sole : Outport  Port=2
  w_H_r_sole : Outport  Port=3
  w_H_rot_task : Outport  Port=4
  w_H_l_hand : Outport  Port=5
  w_H_r_hand : Outport  Port=6
  wires:
  s/1 -> RArm/2, LArm/2, rotational task/2, RFoot/2, LFoot/2, CoM/2
  w_H_b/1 -> RArm/1, LArm/1, rotational task/1, CoM/1, LFoot/1, RFoot/1
  CoM/1 -> w_H_CoM/1
  LFoot/1 -> w_H_l_sole/1
  RFoot/1 -> w_H_r_sole/1
  rotational task/1 -> w_H_rot_task/1
  LArm/1 -> w_H_l_hand/1
  RArm/1 -> w_H_r_hand/1

== system torqueWalking/Robot State and References/State Machines/Compute Feet to Base Link Transforms/LFoot to base link transform /neck transform ==
  neck port : Inport
  Constant : Constant  Value=zeros(3,1)
  Gain : Gain  Gain=pi/180
  Selector1 : Selector  InputPortWidth=6  IndexOptions=Index vector (dialog)  Indices=[1:3]  OutputSizes=1
  Switch : Switch  Criteria=u2 > Threshold
  USE_IMU4EST_BASE1 : Constant  Value=Config.CORRECT_IMU_WITH_NECK_POS
  neck position : Outport
  wires:
  neck port/1 -> Gain/1
  USE_IMU4EST_BASE1/1 -> Switch/2
  Switch/1 -> neck position/1
  Gain/1 -> Selector1/1
  Constant/1 -> Switch/3
  Selector1/1 -> Switch/1  "neck pos"

== system torqueWalking/Robot State and References/State Machines/Compute Feet to Base Link Transforms/RFoot to base link transform/neck transform ==
  neck port : Inport
  Constant : Constant  Value=zeros(3,1)
  Gain : Gain  Gain=pi/180
  Selector1 : Selector  InputPortWidth=6  IndexOptions=Index vector (dialog)  Indices=[1:3]  OutputSizes=1
  Switch : Switch  Criteria=u2 > Threshold
  USE_IMU4EST_BASE1 : Constant  Value=Config.CORRECT_IMU_WITH_NECK_POS
  neck position : Outport
  wires:
  neck port/1 -> Gain/1
  USE_IMU4EST_BASE1/1 -> Switch/2
  Switch/1 -> neck position/1
  Gain/1 -> Selector1/1
  Constant/1 -> Switch/3
  Selector1/1 -> Switch/1  "neck pos"

== matlab function Dynamics and Kinematics/Initial Conditions/compute state velocity/Compute Base Velocity ==
  data: J_LeftFoot input double; J_RightFoot input double; feetInContact input double; nu_b output double; sDot input double; Sat parameter double
function nu_b = computeBaseVelocityFCN(J_LeftFoot, J_RightFoot, feetInContact, sDot, Sat)

    nu_b = computeBaseVelocity(J_LeftFoot, J_RightFoot, feetInContact, sDot, Sat);
end

== matlab function Balancing Controller (Reactive QP control)/Balancing Controller Function ==
  data: feetInContact input double; M input double; Hessian output double; h input double; J input double; impedances input double; dampings input double; s input double; sDot input double; s_sDot_sDDot_des input double; acc_task_star input double; JDot_nu input double; ConstraintsMatrix_feet input double; biasVectorConstraint_feet input double; w_H_l_sole input double; w_H_r_sole input double; gradient output double; ConstraintMatrix_equality output double; biasVectorConstraint_equality output double; ConstraintMatrix_inequality output double; biasVectorConstraint_inequality output double; Sat parameter double; Config parameter double; weights parameter double
function [Hessian,gradient,ConstraintMatrix_equality,biasVectorConstraint_equality, ...
          ConstraintMatrix_inequality,biasVectorConstraint_inequality] = ...
          balancingControllerFCN(feetInContact, M, h, J, impedances, ...
                                 dampings, s, sDot, s_sDot_sDDot_des, acc_task_star, ...
                                 JDot_nu, ConstraintsMatrix_feet, biasVectorConstraint_feet, ...
                                 w_H_l_sole, w_H_r_sole, Sat, Config, weights)
                          

    [Hessian,gradient,ConstraintMatrix_equality,biasVectorConstraint_equality, ...
     ConstraintMatrix_inequality,biasVectorConstraint_inequality] = ...
         balancingControllerMPC(feetInContact, M, h, J, impedances, ...
                                dampings, s, sDot, s_sDot_sDDot_des, acc_task_star, ...
                                JDot_nu, ConstraintsMatrix_feet, biasVectorConstraint_feet, ...
                                w_H_l_sole, w_H_r_sole, Sat, Config, weights);                         
end

== matlab function Dynamics and Kinematics/Inverse Kinematics/Compute tasks accelerations ==
  data: pos_vel_acc_CoM_des input double; acc_task_star output double; pose_vel_acc_LFoot_des input double; pose_vel_acc_RFoot_des input double; orient_vel_acc_rot_task_des input double; pose_vel_acc_LHand_des input double; pose_vel_acc_RHand_des input double; pos_vel_CoM input double; pose_vel_LFoot input double; pose_vel_RFoot input double; orient_vel_rot_task input double; pose_vel_LHand input double; pose_vel_RHand input double; Kp_Kd_CoM input double; Kp_Kd_LFoot input double; Kp_Kd_RFoot input double; Kp_Kd_rot_task input double; Kp_Kd_LHand input double; Kp_Kd_RHand input double; feetInContact input double; Sat parameter double
function acc_task_star = setTasksAccelerationsFCN(pos_vel_acc_CoM_des, pose_vel_acc_LFoot_des, pose_vel_acc_RFoot_des, orient_vel_acc_rot_task_des, pose_vel_acc_LHand_des,pose_vel_acc_RHand_des, ...
                                                  pos_vel_CoM, pose_vel_LFoot, pose_vel_RFoot, orient_vel_rot_task, pose_vel_LHand, pose_vel_RHand, ...
                                                  Kp_Kd_CoM, Kp_Kd_LFoot, Kp_Kd_RFoot, Kp_Kd_rot_task, Kp_Kd_LHand, Kp_Kd_RHand,...
                                                  feetInContact, Sat) 

    acc_task_star = setTasksAccelerations(pos_vel_acc_CoM_des, pose_vel_acc_LFoot_des, pose_vel_acc_RFoot_des, orient_vel_acc_rot_task_des, pose_vel_acc_LHand_des,pose_vel_acc_RHand_des, ...
                                          pos_vel_CoM, pose_vel_LFoot, pose_vel_RFoot, orient_vel_rot_task, pose_vel_LHand, pose_vel_RHand, ...
                                          Kp_Kd_CoM, Kp_Kd_LFoot, Kp_Kd_RFoot, Kp_Kd_rot_task, Kp_Kd_LHand, Kp_Kd_RHand,...
                                          feetInContact, Sat) ; 
                                      
                                      
end

== matlab function Dynamics and Kinematics/Inverse Kinematics/ComputeTasksPoseAndVelocity/Compose Task Pose and Velocity ==
  data: vel_CoM input double; vel_LFoot input double; vel_RFoot input double; vel_rot_task input double; vel_LHand input double; vel_RHand input double; pos_vel_CoM output double; pose_vel_LFoot output double; pose_vel_RFoot output double; orient_vel_rot_task output double; w_H_CoM input double; w_H_l_sole input double; w_H_r_sole input double; w_H_rot_task input double; w_H_l_hand input double; w_H_r_hand input double; pose_vel_LHand output double; pose_vel_RHand output double
function [pos_vel_CoM, pose_vel_LFoot, pose_vel_RFoot, orient_vel_rot_task, pose_vel_LHand, pose_vel_RHand] = ...
             composeTaskPoseAndVelocityFCN(vel_CoM, vel_LFoot, vel_RFoot, vel_rot_task, vel_LHand, vel_RHand, ...
                                           w_H_CoM, w_H_l_sole, w_H_r_sole, w_H_rot_task, w_H_l_hand, w_H_r_hand)
                                                                                                                              
    [pos_vel_CoM, pose_vel_LFoot, pose_vel_RFoot, orient_vel_rot_task, pose_vel_LHand, pose_vel_RHand] = ...
        composeTaskPoseAndVelocity(vel_CoM, vel_LFoot, vel_RFoot, vel_rot_task, vel_LHand, vel_RHand, ...
                                   w_H_CoM, w_H_l_sole, w_H_r_sole, w_H_rot_task, w_H_l_hand, w_H_r_hand);
end

== matlab function Dynamics and Kinematics/Inverse Kinematics/QP-Based Inverse Kinematics/Compute QP Hessian, gradient and constraints  ==
  data: s input double; nu input double; s_sDot_sDDot_ref input double; Hessian output double; impedances input double; dampings input double; J input double; JDot_nu input double; acc_task_star input double; gradient output double; ConstraintMatrix output double; biasVectorConstraint output double
function [Hessian, gradient, ConstraintMatrix, biasVectorConstraint] = ...
             computeQPHessianAndConstraintsFCN(s, nu, s_sDot_sDDot_ref, impedances, dampings, J, JDot_nu, acc_task_star)
    
    %Take off information related to hands tasks -- will not be taken into
    %account for inverse kinematics at this point
    Jtasks = J(1:18,:);
    JDot_nu_tasks = JDot_nu(1:18);
    acc_tasks_star = acc_task_star(1:18);
         
    [Hessian, gradient, ConstraintMatrix, biasVectorConstraint] = ...
        computeQPHessianAndConstraints(s, nu, s_sDot_sDDot_ref, impedances, dampings, Jtasks, JDot_nu_tasks, acc_tasks_star);
end

== matlab function Dynamics and Kinematics/Task Accelerations/Compute tasks accelerations ==
  data: pos_vel_acc_CoM_des input double; acc_task_star output double; pose_vel_acc_LFoot_des input double; pose_vel_acc_RFoot_des input double; orient_vel_acc_rot_task_des input double; pose_vel_acc_LHand_des input double; pose_vel_acc_RHand_des input double; pos_vel_CoM input double; pose_vel_LFoot input double; pose_vel_RFoot input double; orient_vel_rot_task input double; pose_vel_LHand input double; pose_vel_RHand input double; Kp_Kd_CoM input double; Kp_Kd_LFoot input double; Kp_Kd_RFoot input double; Kp_Kd_rot_task input double; Kp_Kd_LHand input double; Kp_Kd_RHand input double; feetInContact input double; Sat parameter double
function acc_task_star = setTasksAccelerationsFCN(pos_vel_acc_CoM_des, pose_vel_acc_LFoot_des, pose_vel_acc_RFoot_des, orient_vel_acc_rot_task_des, pose_vel_acc_LHand_des,pose_vel_acc_RHand_des, ...
                                                  pos_vel_CoM, pose_vel_LFoot, pose_vel_RFoot, orient_vel_rot_task, pose_vel_LHand, pose_vel_RHand, ...
                                                  Kp_Kd_CoM, Kp_Kd_LFoot, Kp_Kd_RFoot, Kp_Kd_rot_task, Kp_Kd_LHand, Kp_Kd_RHand,...
                                                  feetInContact, Sat) 

    acc_task_star = setTasksAccelerations(pos_vel_acc_CoM_des, pose_vel_acc_LFoot_des, pose_vel_acc_RFoot_des, orient_vel_acc_rot_task_des, pose_vel_acc_LHand_des,pose_vel_acc_RHand_des, ...
                                          pos_vel_CoM, pose_vel_LFoot, pose_vel_RFoot, orient_vel_rot_task, pose_vel_LHand, pose_vel_RHand, ...
                                          Kp_Kd_CoM, Kp_Kd_LFoot, Kp_Kd_RFoot, Kp_Kd_rot_task, Kp_Kd_LHand, Kp_Kd_RHand,...
                                          feetInContact, Sat);

end
